simulink model "ControlDiagram"  (R2024a)
settings: Solver=VariableStepAuto  StartTime=0.0  StopTime=10.0  RelTol=1e-3
undefined symbols (not defined in the file): Centroid, FF, Kd, Ki, Kp, V_set
settings Model: Creator=kyle  LastModifiedBy=kyle

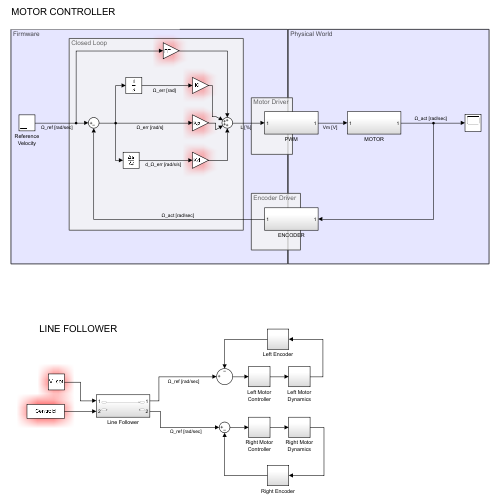
[thumbnail: Simulink's stored preview of the top-level diagram]
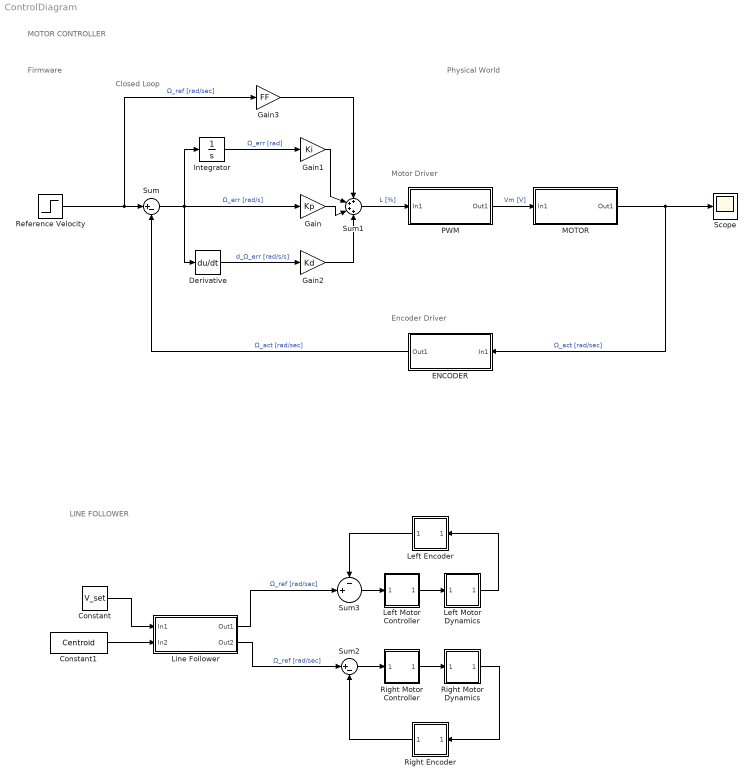
== system ControlDiagram ==
  note: MOTOR CONTROLLER
  note: Encoder Driver
  note: Motor Driver
  note: Closed Loop
  note: Physical World
  note: Firmware
  note: LINE FOLLOWER
  Constant : Constant  Value=V_set
  Constant1 : Constant  Value=Centroid
  Derivative : Derivative
  ENCODER : Subsystem
  Gain : Gain  Gain=Kp
  Gain1 : Gain  Gain=Ki
  Gain2 : Gain  Gain=Kd
  Gain3 : Gain  Gain=FF
  Integrator : Integrator
  Left Encoder : Subsystem
  Left Motor Controller : Subsystem
  Left Motor Dynamics : Subsystem
  Line Follower : Subsystem
  MOTOR : Subsystem
  PWM : Subsystem
  Reference Velocity : Step  SampleTime=0
  Right Encoder : Subsystem
  Right Motor Controller : Subsystem
  Right Motor Dynamics : Subsystem
  Scope : Scope
  Sum : Sum  Inputs=|+-
  Sum1 : Sum  Inputs=++++
  Sum2 : Sum  Inputs=|+-
  Sum3 : Sum  Inputs=-+|
  wires:
  Reference Velocity/1 -> Gain3/1, Sum/1  "Ω_ref [rad/sec]"
  Integrator/1 -> Gain1/1  "Ω_err [rad]"
  Derivative/1 -> Gain2/1  "d_Ω_err [rad/s/s]"
  Sum/1 -> Integrator/1, Derivative/1, Gain/1  "Ω_err [rad/s]"
  Gain/1 -> Sum1/3
  Gain2/1 -> Sum1/4
  Gain1/1 -> Sum1/2
  Sum1/1 -> PWM/1(In1)  "L [%]"
  PWM/1(Out1) -> MOTOR/1(In1)  "Vm [V]"
  MOTOR/1(Out1) -> ENCODER/1(In1), Scope/1  "Ω_act [rad/sec]"
  ENCODER/1(Out1) -> Sum/2  "Ω_act [rad/sec]"
  Gain3/1 -> Sum1/1
  Left Motor Dynamics/1(Out1) -> Left Encoder/1(In1)
  Left Motor Controller/1(Out1) -> Left Motor Dynamics/1(In1)
  Right Motor Dynamics/1(Out1) -> Right Encoder/1(In1)
  Right Motor Controller/1(Out1) -> Right Motor Dynamics/1(In1)
  Constant/1 -> Line Follower/1(In1)
  Constant1/1 -> Line Follower/2(In2)
  Right Encoder/1(Out1) -> Sum2/2
  Sum2/1 -> Right Motor Controller/1(In1)
  Line Follower/2(Out2) -> Sum2/1  "Ω_ref [rad/sec]"
  Sum3/1 -> Left Motor Controller/1(In1)
  Left Encoder/1(Out1) -> Sum3/1
  Line Follower/1(Out1) -> Sum3/2  "Ω_ref [rad/sec]"

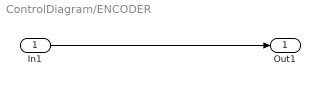
== system ControlDiagram/ENCODER ==
  In1 : Inport
  Out1 : Outport
  wires:
  In1/1 -> Out1/1

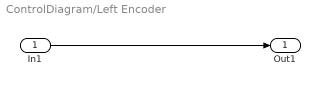
== system ControlDiagram/Left Encoder ==
  In1 : Inport
  Out1 : Outport
  wires:
  In1/1 -> Out1/1

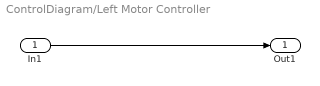
== system ControlDiagram/Left Motor Controller ==
  In1 : Inport
  Out1 : Outport
  wires:
  In1/1 -> Out1/1

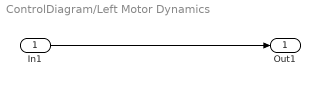
== system ControlDiagram/Left Motor Dynamics ==
  In1 : Inport
  Out1 : Outport
  wires:
  In1/1 -> Out1/1

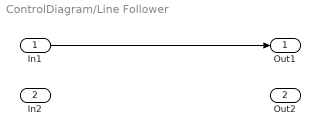
== system ControlDiagram/Line Follower ==
  In1 : Inport
  In2 : Inport  Port=2
  Out1 : Outport
  Out2 : Outport  Port=2
  wires:
  In1/1 -> Out1/1

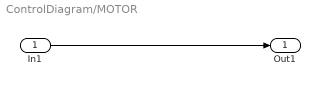
== system ControlDiagram/MOTOR ==
  In1 : Inport
  Out1 : Outport
  wires:
  In1/1 -> Out1/1

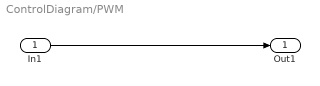
== system ControlDiagram/PWM ==
  In1 : Inport
  Out1 : Outport
  wires:
  In1/1 -> Out1/1

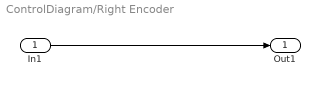
== system ControlDiagram/Right Encoder ==
  In1 : Inport
  Out1 : Outport
  wires:
  In1/1 -> Out1/1

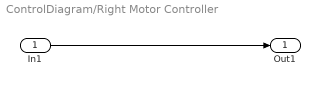
== system ControlDiagram/Right Motor Controller ==
  In1 : Inport
  Out1 : Outport
  wires:
  In1/1 -> Out1/1

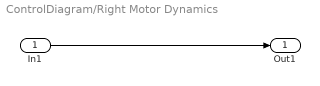
== system ControlDiagram/Right Motor Dynamics ==
  In1 : Inport
  Out1 : Outport
  wires:
  In1/1 -> Out1/1
